simulink model "matrix_mul_transpose"  (R2023b)
settings: Solver=FixedStepAuto  StartTime=0.0  StopTime=10.0  RelTol=1e-3
settings Model: Creator=李骐  LastModifiedBy=李骐
settings OptimizationCC: DefaultParameterBehavior=Inlined  EnhancedBackFolding=on  PassReuseOutputArgsAs=Individual arguments  ZeroExternalMemoryAtStartup=off  ZeroInternalMemoryAtStartup=off  OptimizeBlockOrder=speed  DifferentSizesBufferReuse=on  OptimizationCustomize=off  EfficientTunableParamExpr=on
settings DebuggingCC: ParameterTunabilityLossMsg=error
settings HardwareCC: ProdBitPerLong=64  ProdLongLongMode=on  ProdHWDeviceType=RISC-V->RV64I
settings SFSimCC: MATLABDynamicMemAlloc=off
settings RTWCC: Description=Embedded Coder  SystemTargetFile=ert.tlc  GenCodeOnly=on  TemplateMakefile=ert_default_tmf  TargetLang=C++
settings CodeAppCC: ForceParamTrailComments=on  IgnoreCustomStorageClasses=off  OperatorAnnotations=on  SimulinkDataObjDesc=on  SFDataObjDesc=on  InsertBlockDesc=on
settings ERTTargetCC: TargetLangStandard=C++11 (ISO)  GenerateSampleERTMain=on  CodeInterfacePackaging=C++ class  InlinedParameterPlacement=NonHierarchical  RootIOFormat=Structure reference  ERTCustomFileTemplate=example_file_process.tlc

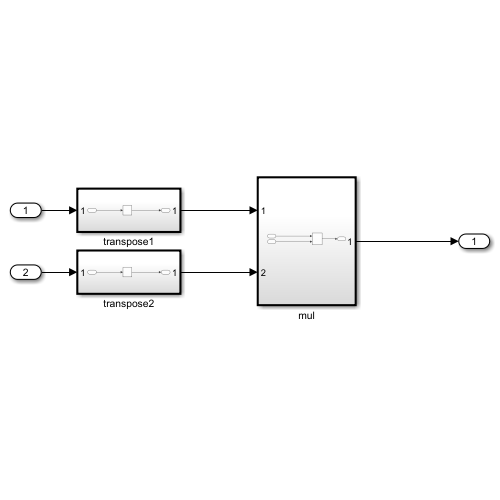
[thumbnail: Simulink's stored preview of the top-level diagram]
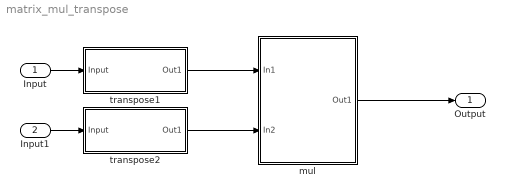
== system matrix_mul_transpose ==
  Input : Inport  PortDimensions=[512 512]
  Input1 : Inport  Port=2  PortDimensions=[512 512]
  mul : Subsystem  TreatAsAtomicUnit=on
      settings: RTWFcnNameOpts=Use subsystem name
  transpose1 : Subsystem  TreatAsAtomicUnit=on
      settings: RTWFcnNameOpts=Use subsystem name
  transpose2 : Subsystem  TreatAsAtomicUnit=on
      settings: RTWFcnNameOpts=Use subsystem name
  Output : Outport
  wires:
  Input/1 -> transpose1/1(Input)
  transpose1/1(Out1) -> mul/1(In1)
  mul/1(Out1) -> Output/1
  Input1/1 -> transpose2/1(Input)
  transpose2/1(Out1) -> mul/2(In2)

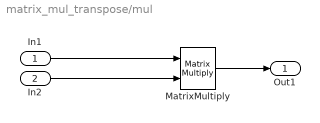
== system matrix_mul_transpose/mul ==
  In1 : Inport
  In2 : Inport  Port=2
  MatrixMultiply : Product  Multiplication=Matrix(*)
  Out1 : Outport
  wires:
  MatrixMultiply/1 -> Out1/1
  In1/1 -> MatrixMultiply/1
  In2/1 -> MatrixMultiply/2

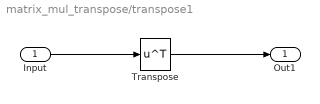
== system matrix_mul_transpose/transpose1 ==
  Input : Inport
  Transpose : Math  Operator=transpose
  Out1 : Outport
  wires:
  Input/1 -> Transpose/1
  Transpose/1 -> Out1/1

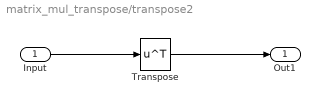
== system matrix_mul_transpose/transpose2 ==
  Input : Inport
  Transpose : Math  Operator=transpose
  Out1 : Outport
  wires:
  Input/1 -> Transpose/1
  Transpose/1 -> Out1/1
